simulink model "Activation_logic"  (R2022b)
settings: Solver=VariableStepAuto  StartTime=0.0  StopTime=10.0  RelTol=1e-3
StartFcn:
  | init
undefined symbols (not defined in the file or in its folder): App_modes
settings Model: Creator=Dell  LastModifiedBy=Dell
settings DataIOCC: ExternalInput=[t, theta]  LoadExternalInput=on  SaveFormat=Array

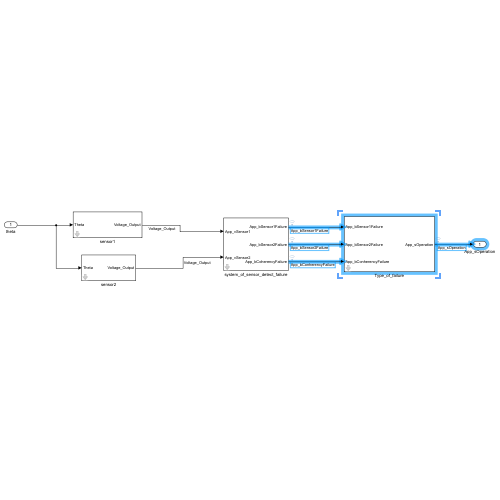
[thumbnail: Simulink's stored preview of the top-level diagram]
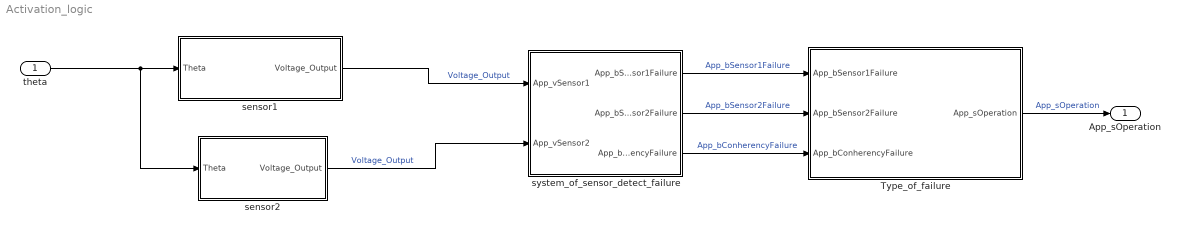
== system Activation_logic ==
  theta : Inport
  Type_of_failure : Subsystem  InitFcn=init
  sensor1 : Subsystem
  sensor2 : Subsystem
  system_of_sensor_detect_failure : Subsystem
  App_sOperation : Outport
  wires:
  Type_of_failure/1(App_sOperation) -> App_sOperation/1  "App_sOperation"
  sensor1/1(Voltage_Output) -> system_of_sensor_detect_failure/1(App_vSensor1)  "Voltage_Output"
  sensor2/1(Voltage_Output) -> system_of_sensor_detect_failure/2(App_vSensor2)  "Voltage_Output"
  theta/1 -> sensor1/1(Theta), sensor2/1(Theta)
  system_of_sensor_detect_failure/1(App_bSensor1Failure) -> Type_of_failure/1(App_bSensor1Failure)  "App_bSensor1Failure"
  system_of_sensor_detect_failure/2(App_bSensor2Failure) -> Type_of_failure/2(App_bSensor2Failure)  "App_bSensor2Failure"
  system_of_sensor_detect_failure/3(App_bCoherencyFailure) -> Type_of_failure/3(App_bConherencyFailure)  "App_bConherencyFailure"

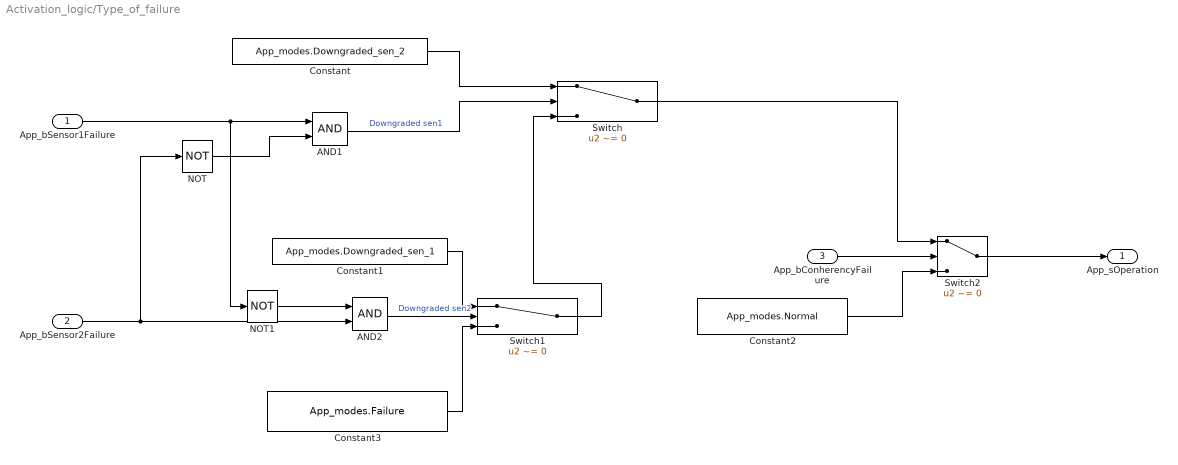
== system Activation_logic/Type_of_failure ==
  App_bSensor1Failure : Inport
  App_bSensor2Failure : Inport  Port=2
  App_bConherencyFailure : Inport  Port=3
  AND1 : Logic  AllPortsSameDT=off  OutDataTypeStr=boolean
  AND2 : Logic  AllPortsSameDT=off  OutDataTypeStr=boolean
  Constant : Constant  Value=App_modes.Downgraded_sen_2  OutDataTypeStr=Enum: App_modes
  Constant1 : Constant  Value=App_modes.Downgraded_sen_1  OutDataTypeStr=Enum: App_modes
  Constant2 : Constant  Value=App_modes.Normal  OutDataTypeStr=Enum: App_modes
  Constant3 : Constant  Value=App_modes.Failure  OutDataTypeStr=Enum: App_modes
  NOT : Logic  Operator=NOT  IconShape=distinctive  AllPortsSameDT=off  OutDataTypeStr=boolean
  NOT1 : Logic  Operator=NOT  IconShape=distinctive  AllPortsSameDT=off  OutDataTypeStr=boolean
  Switch : Switch  Criteria=u2 ~= 0  SaturateOnIntegerOverflow=off  InputSameDT=off
  Switch1 : Switch  Criteria=u2 ~= 0  SaturateOnIntegerOverflow=off  InputSameDT=off
  Switch2 : Switch  Criteria=u2 ~= 0  SaturateOnIntegerOverflow=off  InputSameDT=off
  App_sOperation : Outport  OutDataTypeStr=Enum: App_modes  LockScale=on
  wires:
  NOT/1 -> AND1/2
  NOT1/1 -> AND2/1
  App_bSensor1Failure/1 -> NOT1/1, AND1/1
  App_bSensor2Failure/1 -> NOT/1, AND2/2
  AND1/1 -> Switch/2  "Downgraded sen1"
  AND2/1 -> Switch1/2  "Downgraded sen2"
  Switch/1 -> Switch2/1
  Switch2/1 -> App_sOperation/1
  App_bConherencyFailure/1 -> Switch2/2
  Switch1/1 -> Switch/3
  Constant/1 -> Switch/1
  Constant2/1 -> Switch2/3
  Constant1/1 -> Switch1/1
  Constant3/1 -> Switch1/3

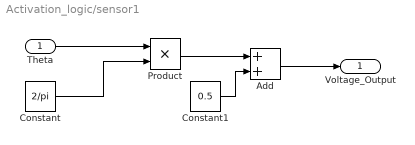
== system Activation_logic/sensor1 ==
  Theta : Inport
  Add : Sum
  Constant : Constant  Value=2/pi
  Constant1 : Constant  Value=0.5
  Product : Product
  Voltage_Output : Outport
  wires:
  Theta/1 -> Product/1
  Add/1 -> Voltage_Output/1
  Constant/1 -> Product/2
  Constant1/1 -> Add/2
  Product/1 -> Add/1

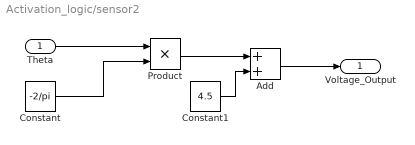
== system Activation_logic/sensor2 ==
  Theta : Inport
  Add : Sum
  Constant : Constant  Value=-2/pi
  Constant1 : Constant  Value=4.5
  Product : Product
  Voltage_Output : Outport
  wires:
  Product/1 -> Add/1
  Constant1/1 -> Add/2
  Constant/1 -> Product/2
  Add/1 -> Voltage_Output/1
  Theta/1 -> Product/1

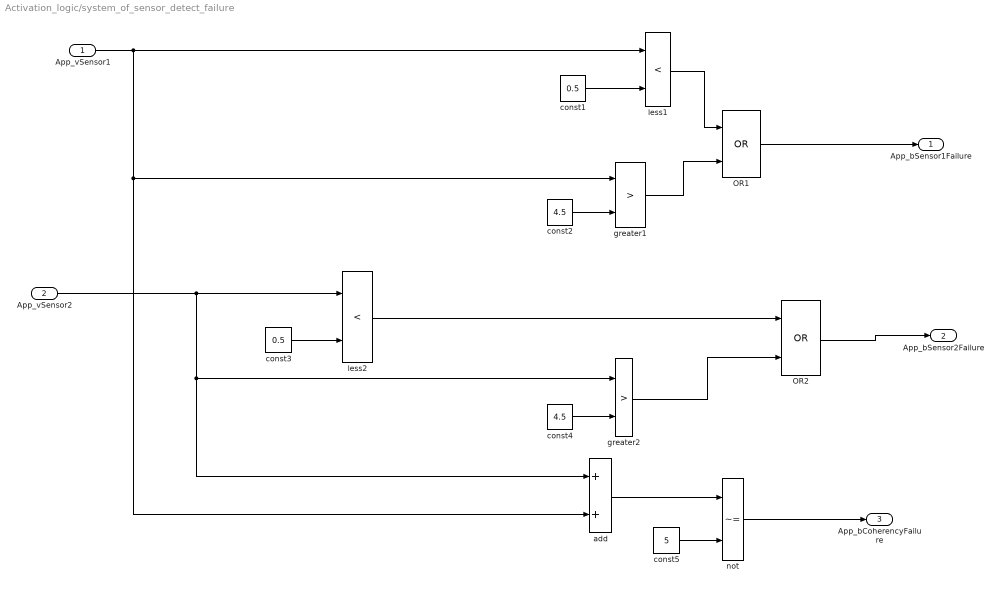
== system Activation_logic/system_of_sensor_detect_failure ==
  App_vSensor1 : Inport
  App_vSensor2 : Inport  Port=2
  OR1 : Logic  Operator=OR  AllPortsSameDT=off  OutDataTypeStr=boolean
  OR2 : Logic  Operator=OR  AllPortsSameDT=off  OutDataTypeStr=boolean
  add : Sum
  const1 : Constant  Value=0.5
  const2 : Constant  Value=4.5
  const3 : Constant  Value=0.5
  const4 : Constant  Value=4.5
  const5 : Constant  Value=5
  greater1 : RelationalOperator  Operator=>  OutDataTypeStr=boolean  RndMeth=Simplest  InputSameDT=off
  greater2 : RelationalOperator  Operator=>  OutDataTypeStr=boolean  RndMeth=Simplest  InputSameDT=off
  less1 : RelationalOperator  Operator=<  OutDataTypeStr=boolean  RndMeth=Simplest  InputSameDT=off
  less2 : RelationalOperator  Operator=<  OutDataTypeStr=boolean  RndMeth=Simplest  InputSameDT=off
  not : RelationalOperator  Operator=~=  OutDataTypeStr=boolean  RndMeth=Simplest  InputSameDT=off
  App_bSensor1Failure : Outport
  App_bSensor2Failure : Outport  Port=2
  App_bCoherencyFailure : Outport  Port=3
  wires:
  App_vSensor1/1 -> less1/1, add/2, greater1/1
  const1/1 -> less1/2
  const2/1 -> greater1/2
  less1/1 -> OR1/1
  greater1/1 -> OR1/2
  OR1/1 -> App_bSensor1Failure/1
  App_vSensor2/1 -> greater2/1, add/1, less2/1
  const3/1 -> less2/2
  const4/1 -> greater2/2
  less2/1 -> OR2/1
  greater2/1 -> OR2/2
  OR2/1 -> App_bSensor2Failure/1
  add/1 -> not/1
  const5/1 -> not/2
  not/1 -> App_bCoherencyFailure/1
